simulink library "Tire_CFL"  (R2023b)
settings: Solver=VariableStepAuto  StartTime=0.0  StopTime=10.0  RelTol=1e-3
undefined symbols (not defined in the file): Tire, Visual
libraries: sm_lib x7, nesl_utility x6, Tire_Utilities x1, TireBody_Systems x1
Description:
  | Component of Simscape Vehicle Templates Library
  | 
  | Copyright 2018-2024 The MathWorks, Inc.
settings Model: Creator=smiller  LastModifiedBy=smiller
settings SolverCC: AlgebraicLoopSolver=TrustRegion
settings DataIOCC: ReturnWorkspaceOutputs=off
settings DebuggingCC: UnconnectedInputMsg=warning  UnconnectedOutputMsg=warning  UnconnectedLineMsg=warning  ArithmeticOperatorsInVariantConditions=warning
settings ModelReferenceCC: EnableRefExpFcnMdlSchedulingChecks=on
settings SFSimCC: CustomCodeUndefinedFunction=UseInterfaceOnly
settings RTWCC: DLArmComputeVersion=19.05

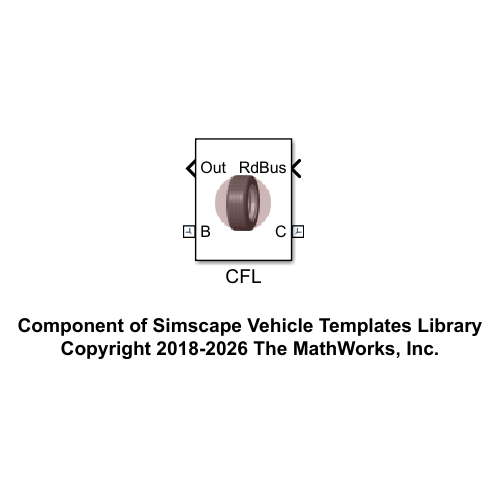
[thumbnail: Simulink's stored preview of the top-level diagram]
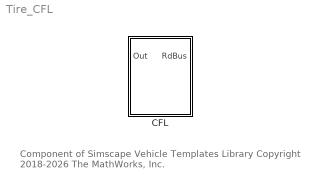
== system Tire_CFL ==
  note: Component of Simscape Vehicle Templates Library
      | Copyright 2018-2026 The MathWorks, Inc.
  CFL : Subsystem  VariantControl=CFL  mask(Tire Model using Spatial Contact Force Block){popup_leftRight=Left, tire_radius=Tire.tire_radius.Value, rim_radius=Tire.rim_radius.Value, tire_width=Tire.tire_width.Value, rim_width=Tire.rim_width.Value, tyre_mass=Tire.tire_mass.Value, rim_mass=Tire.rim_mass.Value, tire_inertia=Tire.tire_J.Value, rim_inertia=Tire.rim_J.Value, plane_l=Tire.plane.l.Value, plane_w=Tire.Plane.w.Value, k_contact=Tire.k.Value, b_contact=Tire.b.Value, mu_kinetic=Tire.mu_k.Value, mu_static=Tire.mu_s.Value, v_thr=Tire.v_thr.Value, TireBody=Tire.TireBody, clr_tyre_cfl=Visual.Tire.clr, opc_tyre_cfl=Visual.Tire.opc, clr_rim_cfl=Visual.Rim.clr, opc_rim_cfl=Visual.Rim.opc}
      mask prompts: popup_leftRight "Left/Right"; plane_l "Plane Length (m)"; plane_w "Plane Width (m)"; k_contact "Stiffness (N/m)"; b_contact "Damping (N/(m/s))"; mu_kinetic "Coefficient of Kinetic Friction"; mu_static "Coefficient of Static Friction"; v_thr "Velocity Threshold (m/s)"; TireBody "Tire Body (structure)"
      mask help: Models a tire using the Spatial Contact Force Block. A sphere is used for the contact geometry. The default contact force law is used for contact with the ground. For very simple, low speed tests only.
      mask init:
      | tyre_Ixx = tire_inertia(1);
      | tyre_Iyy = tire_inertia(2);
      | 
      | curblk = gcb;
      | 
      | if(popup_leftRight == 1)
      |     set_param([gcb '/Tire Body'],'popup_leftRight','Left');
      | elseif(popup_leftRight == 2)
      |     set_param([gcb '/Tire Body'],'popup_leftRight','Right');
      | end
      mask TypeOptions popup_leftRight: Left | Right
      mask TypeOptions k_contact: Tire and Force/k_contact
      mask TypeOptions b_contact: Tire and Force/b_contact
      mask TypeOptions mu_kinetic: Tire and Force/mu_kinetic
      mask TypeOptions mu_static: Tire and Force/mu_static
      mask TypeOptions v_thr: Tire and Force/v_thr
      mask TypeOptions clr_tyre_cfl: Tire and Force/clr_tyre_cfl
      mask TypeOptions opc_tyre_cfl: Tire and Force/opc_tyre_cfl
      mask TypeOptions clr_rim_cfl: Tire and Force/clr_rim_cfl
      mask TypeOptions opc_rim_cfl: Tire and Force/opc_rim_cfl
      mask DialogControl cont_tyre_cfl Prompt: Contact Force Tire
      mask DialogControl group_tire_dim Prompt: Dimensions
      mask DialogControl text_tire_tire Prompt: Tire
      mask DialogControl text_tire_rim Prompt: Rim
      mask DialogControl text_tire_dim_radius Prompt: Radius (m)
      mask DialogControl text_tire_dim_width Prompt: Width (m)
      mask DialogControl text_tire_mass Prompt: Mass (kg)
      mask DialogControl text_tire_inertia Prompt: Inertia [Ixx Iyy]
      mask DialogControl group_tyre_cflkb Prompt: Contact
      mask DialogControl cont_tire_cfl_vis Prompt: Visualization
      mask DialogControl text_vis_tire_cfl_clr Prompt: Color [RGB]
      mask DialogControl text_vis_tire_cfl_opc Prompt: Opacity (0-1)
      mask DialogControl text_vis_tire_tyre Prompt: Tyre
      mask DialogControl text_vis_tire_rim Prompt: Rim
      mask Display: image('sm_car_vehicle_tire_cfl_IMAGE.png');

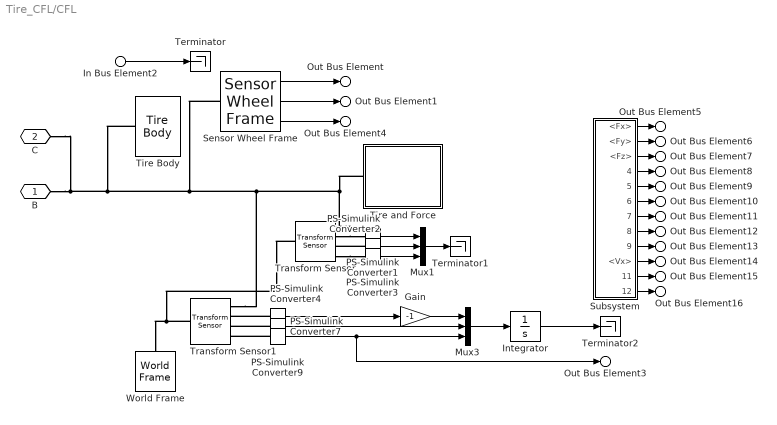
== system Tire_CFL/CFL ==
  In Bus Element2 : Inport  PortName=RdBus  Element=gz
  Gain : Gain  Gain=-1
  Integrator : Integrator  WrapState=on  WrappedStateUpperValue=2*pi  WrappedStateLowerValue=0
  Mux1 : Mux  Inputs=3
  Mux3 : Mux  Inputs=3
  PS-Simulink Converter1 : nesl_utility/PS-Simulink Converter  PhysicalDomain=network_engine_domain  SubClassName=ps_output  LeftPortType=input  RightPortType=output  PseudoPeriodic=off  Frequencies=[]  VectorFormat=1-D array  Unit=m  AffineConversion=off
  PS-Simulink Converter2 : nesl_utility/PS-Simulink Converter  PhysicalDomain=network_engine_domain  SubClassName=ps_output  LeftPortType=input  RightPortType=output  PseudoPeriodic=off  Frequencies=[]  VectorFormat=1-D array  Unit=1  AffineConversion=off
  PS-Simulink Converter3 : nesl_utility/PS-Simulink Converter  PhysicalDomain=network_engine_domain  SubClassName=ps_output  LeftPortType=input  RightPortType=output  PseudoPeriodic=off  Frequencies=[]  VectorFormat=1-D array  Unit=1  AffineConversion=off
  PS-Simulink Converter4 : nesl_utility/PS-Simulink Converter  PhysicalDomain=network_engine_domain  SubClassName=ps_output  LeftPortType=input  RightPortType=output  PseudoPeriodic=off  Frequencies=[]  VectorFormat=1-D array  Unit=rad/s  AffineConversion=off
  PS-Simulink Converter7 : nesl_utility/PS-Simulink Converter  PhysicalDomain=network_engine_domain  SubClassName=ps_output  LeftPortType=input  RightPortType=output  PseudoPeriodic=off  Frequencies=[]  VectorFormat=1-D array  Unit=rad/s  AffineConversion=off
  PS-Simulink Converter9 : nesl_utility/PS-Simulink Converter  PhysicalDomain=network_engine_domain  SubClassName=ps_output  LeftPortType=input  RightPortType=output  PseudoPeriodic=off  Frequencies=[]  VectorFormat=1-D array  Unit=rad/s  AffineConversion=off
  Sensor Wheel Frame : Tire_Utilities/Sensor Wheel Frame  SystemSampleTime=-1  VariantActivationTime=update diagram  AllowFlexibleInterface=on  Latency=0  AutoFrameSizeCalculation=off
  Subsystem : Subsystem
  Terminator : Terminator
  Terminator1 : Terminator
  Terminator2 : Terminator
  Tire Body : TireBody_Systems/Tire Body  LabelModeActiveChoice=Parameterized  popup_leftRight=Right  TireBody=TireBody  VariantLabel=TireBody.class.Value
  Tire and Force : Subsystem  mask{tire_radius=tire_radius, plane_l=plane_l, plane_w=plane_w, NormalStiffness=k_contact, NormalDamping=b_contact, CoefficientOfDynamicFriction=mu_static, CoefficientOfStaticFriction=mu_kinetic, FrictionalCriticalVelocity=v_thr}
      mask prompts: tire_radius "Tire Radius (m)"; plane_l "Plane Length (m)"; plane_w "Plane Width (m)"; NormalStiffness "Stiffness (N/m)"; NormalDamping "Damping (N/(m/s))"; CoefficientOfDynamicFriction "Coefficient of Kinetic Friction"; CoefficientOfStaticFriction "Coefficient of Static Friction"; FrictionalCriticalVelocity "Velocity Threshold (m/s)"
      mask TypeOptions NormalStiffness:
      | Spatial
      | Contact Force/NormalStiffness
      mask TypeOptions NormalDamping:
      | Spatial
      | Contact Force/NormalDamping
      mask TypeOptions CoefficientOfDynamicFriction:
      | Spatial
      | Contact Force/CoefficientOfDynamicFriction
      mask TypeOptions CoefficientOfStaticFriction:
      | Spatial
      | Contact Force/CoefficientOfStaticFriction
      mask TypeOptions FrictionalCriticalVelocity:
      | Spatial
      | Contact Force/FrictionalCriticalVelocity
      mask DialogControl cont_tyre_cfl Prompt: Contact Force Tyre
      mask DialogControl group_tyre_dim Prompt: Dimensions
      mask DialogControl group_tyre_cflkb Prompt: Contact
  Transform Sensor : sm_lib/Frames and Transforms/Transform Sensor  MeasurementFrame=World  RotationSequence=XYX  SenseAngle=off  SenseAxis=off  SenseQ=off  SenseR=off  SenseRotationSequence=off  SenseOmegaX=off  SenseOmegaY=off  SenseOmegaZ=off  SenseOmega=off  SenseQDot=off  SenseRDot=off  SenseRotationSequenceDot=off  SenseAlphaX=off  SenseAlphaY=off  SenseAlphaZ=off  SenseAlpha=off  SenseQDDot=off  SenseRDDot=off  SenseX=on  SenseY=on  SenseZ=on  SenseXYZ=off  SenseRad=off  SenseAzim=off  SenseDist=off  SenseInc=off  SenseXDot=off  SenseYDot=off  SenseZDot=off  SenseXYZDot=off  SenseRadDot=off  SenseAzimDot=off  SenseDistDot=off  SenseIncDot=off  SenseXDDot=off  SenseYDDot=off  SenseZDDot=off  SenseXYZDDot=off  SenseRadDDot=off  SenseAzimDDot=off  SenseDistDDot=off  SenseIncDDot=off
  Transform Sensor1 : sm_lib/Frames and Transforms/Transform Sensor  MeasurementFrame=NonRotatingFollower  RotationSequence=XYX  SenseAngle=off  SenseAxis=off  SenseQ=off  SenseR=off  SenseRotationSequence=off  SenseOmegaX=on  SenseOmegaY=on  SenseOmegaZ=on  SenseOmega=off  SenseQDot=off  SenseRDot=off  SenseRotationSequenceDot=off  SenseAlphaX=off  SenseAlphaY=off  SenseAlphaZ=off  SenseAlpha=off  SenseQDDot=off  SenseRDDot=off  SenseX=off  SenseY=off  SenseZ=off  SenseXYZ=off  SenseRad=off  SenseAzim=off  SenseDist=off  SenseInc=off  SenseXDot=off  SenseYDot=off  SenseZDot=off  SenseXYZDot=off  SenseRadDot=off  SenseAzimDot=off  SenseDistDot=off  SenseIncDot=off  SenseXDDot=off  SenseYDDot=off  SenseZDDot=off  SenseXYZDDot=off  SenseRadDDot=off  SenseAzimDDot=off  SenseDistDDot=off  SenseIncDDot=off
  World Frame : sm_lib/Frames and Transforms/World Frame
  B : PMIOPort  Side=Right
  C : PMIOPort  Port=2  Side=Left
  Out Bus Element3 : Outport  VectorParamsAs1DForOutWhenUnconnected=off  PortName=Out  Element=omega
  Out Bus Element : Outport  VectorParamsAs1DForOutWhenUnconnected=off  PortName=Out  Element=qxyz
  Out Bus Element1 : Outport  VectorParamsAs1DForOutWhenUnconnected=off  PortName=Out  Element=xyz
  Out Bus Element4 : Outport  VectorParamsAs1DForOutWhenUnconnected=off  PortName=Out  Element=n
  Out Bus Element5 : Outport  VectorParamsAs1DForOutWhenUnconnected=off  PortName=Out  Element=Fx
  Out Bus Element6 : Outport  VectorParamsAs1DForOutWhenUnconnected=off  PortName=Out  Element=Fy
  Out Bus Element7 : Outport  VectorParamsAs1DForOutWhenUnconnected=off  PortName=Out  Element=Fz
  Out Bus Element8 : Outport  VectorParamsAs1DForOutWhenUnconnected=off  PortName=Out  Element=Mx
  Out Bus Element9 : Outport  VectorParamsAs1DForOutWhenUnconnected=off  PortName=Out  Element=My
  Out Bus Element10 : Outport  VectorParamsAs1DForOutWhenUnconnected=off  PortName=Out  Element=Mz
  Out Bus Element11 : Outport  VectorParamsAs1DForOutWhenUnconnected=off  PortName=Out  Element=rSlip
  Out Bus Element12 : Outport  VectorParamsAs1DForOutWhenUnconnected=off  PortName=Out  Element=aSlip
  Out Bus Element13 : Outport  VectorParamsAs1DForOutWhenUnconnected=off  PortName=Out  Element=aCamber
  Out Bus Element14 : Outport  VectorParamsAs1DForOutWhenUnconnected=off  PortName=Out  Element=vx
  Out Bus Element15 : Outport  VectorParamsAs1DForOutWhenUnconnected=off  PortName=Out  Element=rMuX
  Out Bus Element16 : Outport  VectorParamsAs1DForOutWhenUnconnected=off  PortName=Out  Element=rMuY
  wires:
  PS-Simulink Converter7/1 -> Mux3/2
  PS-Simulink Converter4/1 -> Gain/1
  Mux3/1 -> Integrator/1
  Integrator/1 -> Terminator2/1
  PS-Simulink Converter9/1 -> Out Bus Element3/1, Mux3/3
  PS-Simulink Converter1/1 -> Mux1/1
  PS-Simulink Converter2/1 -> Mux1/2
  Mux1/1 -> Terminator1/1
  Gain/1 -> Mux3/1
  PS-Simulink Converter3/1 -> Mux1/3
  In Bus Element2/1 -> Terminator/1
  Sensor Wheel Frame/3 -> Out Bus Element4/1
  Sensor Wheel Frame/2 -> Out Bus Element1/1
  Sensor Wheel Frame/1 -> Out Bus Element/1
  Subsystem/7(<longitudinal_slip>) -> Out Bus Element11/1
  Subsystem/3(<Fz>) -> Out Bus Element7/1
  Subsystem/12(<mu_y>) -> Out Bus Element16/1
  Subsystem/2(<Fy>) -> Out Bus Element6/1
  Subsystem/9(<inclination_angle>) -> Out Bus Element13/1
  Subsystem/10(<Vx>) -> Out Bus Element14/1
  Subsystem/6(<Mz>) -> Out Bus Element10/1
  Subsystem/8(<side_slip_angle>) -> Out Bus Element12/1
  Subsystem/11(<mu_x>) -> Out Bus Element15/1
  Subsystem/4(<Mx>) -> Out Bus Element8/1
  Subsystem/5(<My>) -> Out Bus Element9/1
  Subsystem/1(<Fx>) -> Out Bus Element5/1
  connections:
  Tire and Force/LConn1 -- Transform Sensor/RConn1 -- Sensor Wheel Frame/LConn1 -- Tire Body/LConn1 -- C/RConn1 -- B/RConn1 -- Transform Sensor1/RConn1
  PS-Simulink Converter9/LConn1 -- Transform Sensor1/RConn4
  Transform Sensor1/LConn1 -- Transform Sensor/LConn1 -- World Frame/RConn1
  PS-Simulink Converter7/LConn1 -- Transform Sensor1/RConn3
  Transform Sensor/RConn2 -- PS-Simulink Converter1/LConn1
  PS-Simulink Converter2/LConn1 -- Transform Sensor/RConn3
  Transform Sensor/RConn4 -- PS-Simulink Converter3/LConn1
  PS-Simulink Converter4/LConn1 -- Transform Sensor1/RConn2

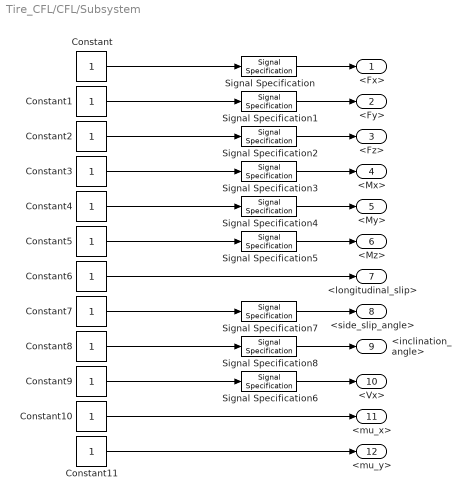
== system Tire_CFL/CFL/Subsystem ==
  Constant{,1..11} (12 alike) : Constant
  Signal Specification : SignalSpecification  Unit=N
  Signal Specification1 : SignalSpecification  Unit=N
  Signal Specification2 : SignalSpecification  Unit=N
  Signal Specification3 : SignalSpecification  Unit=N*m
  Signal Specification4 : SignalSpecification  Unit=N*m
  Signal Specification5 : SignalSpecification  Unit=N*m
  Signal Specification6 : SignalSpecification  Unit=m/s
  Signal Specification7 : SignalSpecification  Unit=rad
  Signal Specification8 : SignalSpecification  Unit=rad
  <Fx> : Outport  VectorParamsAs1DForOutWhenUnconnected=off
  <Fy> : Outport  Port=2  VectorParamsAs1DForOutWhenUnconnected=off
  <Fz> : Outport  Port=3  VectorParamsAs1DForOutWhenUnconnected=off
  <Mx> : Outport  Port=4  VectorParamsAs1DForOutWhenUnconnected=off
  <My> : Outport  Port=5  VectorParamsAs1DForOutWhenUnconnected=off
  <Mz> : Outport  Port=6  VectorParamsAs1DForOutWhenUnconnected=off
  <longitudinal_slip> : Outport  Port=7  VectorParamsAs1DForOutWhenUnconnected=off
  <side_slip_angle> : Outport  Port=8  VectorParamsAs1DForOutWhenUnconnected=off
  <inclination_angle> : Outport  Port=9  VectorParamsAs1DForOutWhenUnconnected=off
  <Vx> : Outport  Port=10  VectorParamsAs1DForOutWhenUnconnected=off
  <mu_x> : Outport  Port=11  VectorParamsAs1DForOutWhenUnconnected=off
  <mu_y> : Outport  Port=12  VectorParamsAs1DForOutWhenUnconnected=off
  wires:
  Constant8/1 -> Signal Specification8/1
  Constant9/1 -> Signal Specification6/1
  Constant1/1 -> Signal Specification1/1
  Constant3/1 -> Signal Specification3/1
  Constant2/1 -> Signal Specification2/1
  Constant10/1 -> <mu_x>/1
  Constant5/1 -> Signal Specification5/1
  Constant/1 -> Signal Specification/1
  Constant7/1 -> Signal Specification7/1
  Constant4/1 -> Signal Specification4/1
  Constant6/1 -> <longitudinal_slip>/1
  Constant11/1 -> <mu_y>/1
  Signal Specification/1 -> <Fx>/1
  Signal Specification1/1 -> <Fy>/1
  Signal Specification2/1 -> <Fz>/1
  Signal Specification3/1 -> <Mx>/1
  Signal Specification4/1 -> <My>/1
  Signal Specification5/1 -> <Mz>/1
  Signal Specification6/1 -> <Vx>/1
  Signal Specification7/1 -> <side_slip_angle>/1
  Signal Specification8/1 -> <inclination_angle>/1

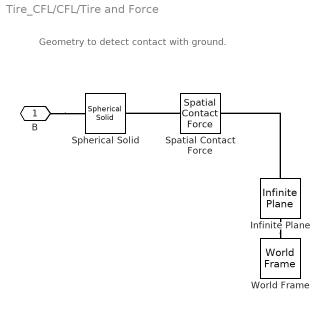
== system Tire_CFL/CFL/Tire and Force ==
  note: Geometry to detect contact with ground.
  Infinite Plane : sm_lib/Curves and Surfaces/Infinite Plane  GraphicType=Rectangle  GraphicPlaneWidth=1  GraphicPlaneWidthUnits=m  GraphicPlaneHeight=1  GraphicPlaneHeightUnits=m  GraphicVisPropType=SimpleVisualProperties  GraphicDiffuseColor=[0.5 0.5 0.5]  GraphicOpacity=0.25  GraphicSpecularColor=[0.5 0.5 0.5 1.0]  GraphicAmbientColor=[0.15 0.15 0.15 1.0]  GraphicEmissiveColor=[0.0 0.0 0.0 1.0]  GraphicShininess=75
  Spatial Contact Force : sm_lib/Forces and Torques/Spatial Contact Force  SenseContactBaseRotation=off  SenseContactBaseTranslation=off  CoefficientOfDynamicFriction=CoefficientOfDynamicFriction  CoefficientOfStaticFriction=CoefficientOfStaticFriction  NormalDamping=NormalDamping  NormalDampingUnits=N/(m/s)  SenseContactSignal=off  NormalStiffness=NormalStiffness  NormalStiffnessUnits=N/m  FrictionalCriticalVelocity=FrictionalCriticalVelocity  FrictionalCriticalVelocityUnits=m/s  ZeroCrossDetectContactStartAndEnd=off  SenseContactFollowerRotation=off  SenseContactFollowerTranslation=off  FrictionType=SmoothStickSlip  SenseFrictionalForceMagnitude=off  SenseNormalForceMagnitude=off  NormalForceType=SmoothSpringDamper  SenseNormalVelocity=off  SensePenetrationDepth=off  SenseSeparationDistance=off  SenseTangentialVelocity=off  NormalTransitionRegionWidth=1e-2  NormalTransitionRegionWidthUnits=m
  Spherical Solid : sm_lib/Body Elements/Spherical Solid  GraphicAmbientColor=[0.15 0.15 0.15 1.0]  BasedOnType=Density  CenterOfMass=[0 0 0]  CenterOfMassUnits=m  GraphicDiffuseColor=[0.5 0.5 0.5]  Density=1000  DensityUnits=kg/m^3  DoExposeReferenceFrame=on  GraphicEmissiveColor=[0.0 0.0 0.0 1.0]  ExportEntireGeometry=on  SerializedExposedGeometries=<ExposedGeometries><ExposedGeometry><RawGeometryId>entire</RawGeometryId><ExposedGeometryId>G</ExposedGeometryId></ExposedGeometry></ExposedGeometries>  SerializedFrames=<Frames/>  MarkerShape=Sphere  MarkerSize=10  GraphicType=None  InertiaType=PointMass  Mass=0  MassUnits=kg  MomentsOfInertia=[1 1 1]  MomentsOfInertiaUnits=kg*m^2  GraphicOpacity=1.0  ProductsOfInertia=[0 0 0]  ProductsOfInertiaUnits=kg*m^2  GraphicShininess=75  GraphicSpecularColor=[0.5 0.5 0.5 1.0]  SphereRadius=tire_radius  SphereRadiusUnits=m  GraphicVisPropType=SimpleVisualProperties
  World Frame : sm_lib/Frames and Transforms/World Frame
  B : PMIOPort  Side=Left
  connections:
  B/RConn1 -- Spherical Solid/RConn1
  Infinite Plane/LConn1 -- World Frame/RConn1
  Spatial Contact Force/RConn1 -- Spherical Solid/LConn1
  Infinite Plane/RConn1 -- Spatial Contact Force/LConn1
